simulink model "model_c"  (R2020a)
settings: Solver=VariableStepAuto  StartTime=0.0  StopTime=10.0  RelTol=1e-3
values from neighbouring files (symbols this model uses):
  c1 = 100    [ode45_b.m]    (also in ode45_c.m; parameters.m)
  c2 = 1000    [ode45_b.m]    (also in ode45_c.m; parameters.m)
  k1 = 10000    [ode45_b.m]    (also in ode45_c.m; parameters.m)
  k2 = 100000    [ode45_b.m]    (also in ode45_c.m; parameters.m)
  m1 = 10    [ode45_b.m]    (also in ode45_c.m; parameters.m)
  m2 = 100    [ode45_b.m]    (also in ode45_c.m; parameters.m)
settings Model: Creator=DEVESH  LastModifiedBy=DEVESH

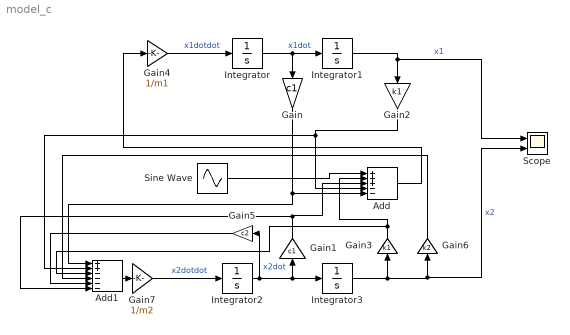
== system model_c ==
  Add : Sum  Inputs=+++--
  Add1 : Sum  Inputs=++----
  Gain : Gain  Gain=c1
  Gain1 : Gain  Gain=c1
  Gain2 : Gain  Gain=k1
  Gain3 : Gain  Gain=k1
  Gain4 : Gain  Gain=1/m1
  Gain5 : Gain  Gain=c2
  Gain6 : Gain  Gain=k2
  Gain7 : Gain  Gain=1/m2
  Integrator{,1..3} (4 alike) : Integrator
  Scope : Scope  NumInputPorts=2
  Sine Wave : Sin  Amplitude=3  Frequency=10  SampleTime=0
  wires:
  Integrator2/1 -> Gain5/1, Gain1/1, Integrator3/1  "x2dot"
  Integrator/1 -> Integrator1/1, Gain/1  "x1dot"
  Gain6/1 -> Add1/4
  Gain5/1 -> Add1/5
  Gain3/1 -> Add1/3, Add/2
  Gain/1 -> Add1/1, Add/5
  Sine Wave/1 -> Add/1
  Gain2/1 -> Add1/2, Add/4
  Gain7/1 -> Integrator2/1  "x2dotdot"
  Add1/1 -> Gain7/1
  Gain1/1 -> Add1/6, Add/3
  Integrator1/1 -> Scope/1, Gain2/1  "x1"
  Integrator3/1 -> Scope/2, Gain6/1, Gain3/1  "x2"
  Add/1 -> Gain4/1
  Gain4/1 -> Integrator/1  "x1dotdot"
